simulink model "ex4_7"  (R2022b)
settings: Solver=FixedStepAuto  StartTime=0.0  StopTime=100  FixedStep=0.01  RelTol=1e-3
settings Model: Creator=13322  LastModifiedBy=31883
settings DebuggingCC: UnconnectedInputMsg=warning  UnconnectedOutputMsg=warning  UnconnectedLineMsg=warning
settings ModelReferenceCC: EnableRefExpFcnMdlSchedulingChecks=on
settings RTWCC: DLArmComputeVersion=19.05

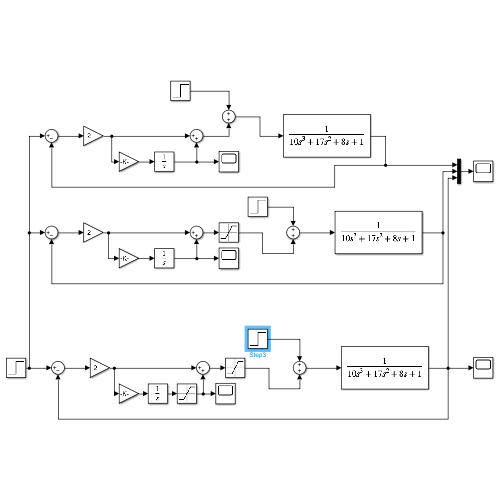
[thumbnail: Simulink's stored preview of the top-level diagram]
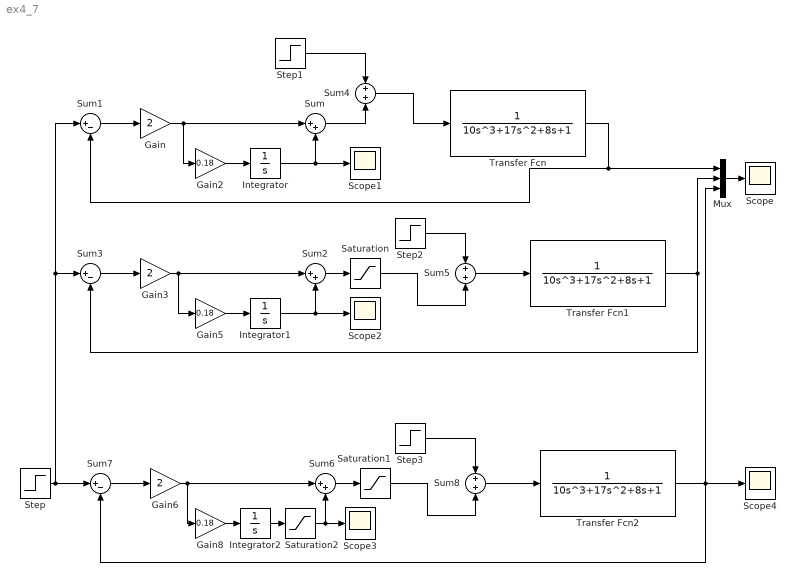
== system ex4_7 ==
  Gain : Gain  Gain=2
  Gain2 : Gain  Gain=0.18
  Gain3 : Gain  Gain=2
  Gain5 : Gain  Gain=0.18
  Gain6 : Gain  Gain=2
  Gain8 : Gain  Gain=0.18
  Integrator : Integrator
  Integrator1 : Integrator
  Integrator2 : Integrator
  Mux : Mux  Inputs=3
  Saturation : Saturate  UpperLimit=1.2  LowerLimit=-1.2
  Saturation1 : Saturate  UpperLimit=1.5  LowerLimit=-1.5
  Saturation2 : Saturate  UpperLimit=0.8  LowerLimit=-0.8
  Scope{,1..4} (5 alike) : Scope
  Step : Step  Time=5  SampleTime=0
  Step1 : Step  Time=50  After=2.5  SampleTime=0
  Step2 : Step  Time=50  After=2.5  SampleTime=0
  Step3 : Step  Time=50  After=2.5  SampleTime=0
  Sum : Sum  Inputs=|++
  Sum1 : Sum  Inputs=|+-
  Sum2 : Sum  Inputs=|++
  Sum3 : Sum  Inputs=|+-
  Sum4 : Sum
  Sum5 : Sum
  Sum6 : Sum  Inputs=|++
  Sum7 : Sum  Inputs=|+-
  Sum8 : Sum
  Transfer Fcn : TransferFcn  Denominator=[10 17 8 1]
  Transfer Fcn1 : TransferFcn  Denominator=[10 17 8 1]
  Transfer Fcn2 : TransferFcn  Denominator=[10 17 8 1]
  wires:
  Gain2/1 -> Integrator/1
  Gain/1 -> Gain2/1, Sum/1
  Integrator/1 -> Scope1/1, Sum/2
  Sum1/1 -> Gain/1
  Transfer Fcn/1 -> Sum1/2, Mux/1
  Sum3/1 -> Gain3/1
  Integrator1/1 -> Scope2/1, Sum2/2
  Gain5/1 -> Integrator1/1
  Transfer Fcn1/1 -> Sum3/2, Mux/2
  Gain3/1 -> Gain5/1, Sum2/1
  Sum2/1 -> Saturation/1
  Mux/1 -> Scope/1
  Sum4/1 -> Transfer Fcn/1
  Sum/1 -> Sum4/2
  Step1/1 -> Sum4/1
  Step2/1 -> Sum5/1
  Saturation/1 -> Sum5/2
  Sum5/1 -> Transfer Fcn1/1
  Transfer Fcn2/1 -> Scope4/1, Sum7/2, Mux/3
  Gain8/1 -> Integrator2/1
  Gain6/1 -> Gain8/1, Sum6/1
  Step/1 -> Sum1/1, Sum3/1, Sum7/1
  Sum6/1 -> Saturation1/1
  Sum7/1 -> Gain6/1
  Sum8/1 -> Transfer Fcn2/1
  Saturation1/1 -> Sum8/2
  Step3/1 -> Sum8/1
  Integrator2/1 -> Saturation2/1
  Saturation2/1 -> Scope3/1, Sum6/2
